simulink model "lqr_pos_control"  (R2021a)
settings: Solver=FixedStepAuto  StartTime=0.0  StopTime=inf  FixedStep=.01  RelTol=1e-3
model workspace (MAT data in the model file):
  SL_ROS_VariableLengthArrays_MaxSizes : object (value not decoded)
values from neighbouring files (symbols this model uses):
  airframe = struct()    [discreteModel_initializer.m]
  Fs = 100    [discreteModel_initializer.m]
  g = 9.81    [discreteModel_initializer.m]
  kLQR = dlqr(lqrDiscrete.A,lqrDiscrete.B,Q,R)    [discreteModel_initializer.m]
  Ts = 1/Fs    (= 0.01)    [discreteModel_initializer.m]
  wiHover = sqrt(((airframe.mass)*9.81)/(4*airframe.Propeller.Ct))    [discreteModel_initializer.m]
undefined symbols (not defined in the file or in its folder): DiscIntNeverNeededParam, Discrete, Gyro_pitch, Gyro_roll, P00, P01, P11, Qkalman, Rkalman, RPM_to_DC, rpmKnown_throttleUnknown, sigbuilder_block, tf1, Time
libraries: robotlib x11, arduinolib x6, sharedtransform x3, simulink x3, ctrlSharedLib x1
(part 2 of 2)

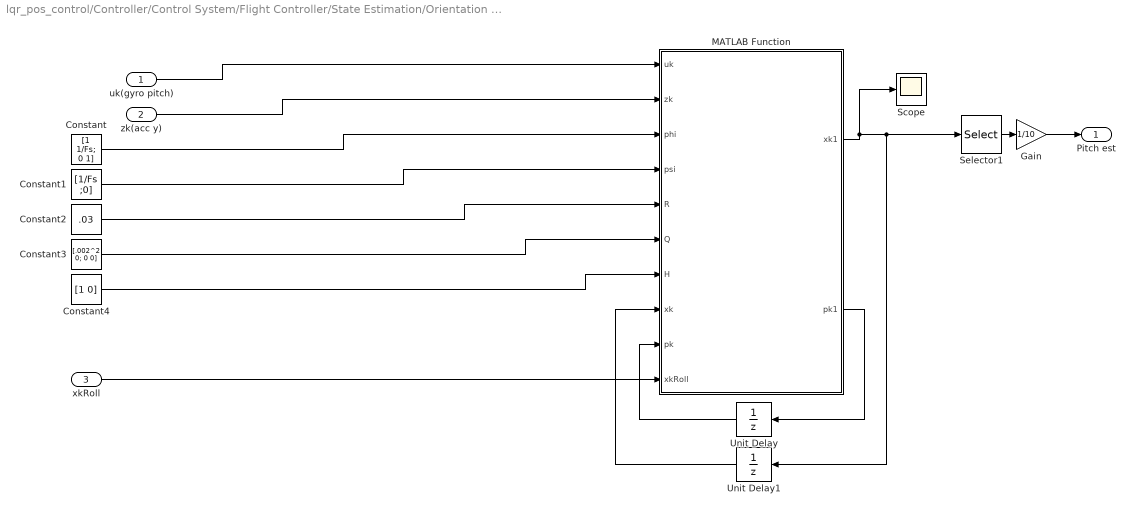
== system lqr_pos_control/Controller/Control System/Flight Controller/State Estimation/Orientation Estimation/Kalman/Kalman Pitch ==
  uk(gyro pitch) : Inport
  zk(acc y) : Inport  Port=2
  xkRoll : Inport  Port=3
  Constant : Constant  Value=[1 1/Fs; 0 1]
  Constant1 : Constant  Value=[1/Fs ;0]
  Constant2 : Constant  Value=.03
  Constant3 : Constant  Value=[.002^2 0; 0 0]
  Constant4 : Constant  Value=[1 0]
  Gain : Gain  Gain=1/10
  MATLAB Function : MATLAB Function  TreatAsAtomicUnit=on
  Scope : Scope
  Selector1 : Selector  InputPortWidth=2  IndexOptions=Index vector (dialog)  Indices=1  OutputSizes=1
  Unit Delay : UnitDelay  InitialCondition=[.5 0; 0 0.01]  SampleTime=-1  HasFrameUpgradeWarning=on
  Unit Delay1 : UnitDelay  InitialCondition=[0;0]  SampleTime=-1  HasFrameUpgradeWarning=on
  Pitch est : Outport
  wires:
  MATLAB Function/1(xk1) -> Scope/1, Unit Delay1/1, Selector1/1
  uk(gyro pitch)/1 -> MATLAB Function/1(uk)
  zk(acc y)/1 -> MATLAB Function/2(zk)
  Constant/1 -> MATLAB Function/3(phi)
  Constant1/1 -> MATLAB Function/4(psi)
  Constant2/1 -> MATLAB Function/5(R)
  Constant3/1 -> MATLAB Function/6(Q)
  Constant4/1 -> MATLAB Function/7(H)
  Selector1/1 -> Gain/1
  Gain/1 -> Pitch est/1
  xkRoll/1 -> MATLAB Function/10(xkRoll)
  MATLAB Function/2(pk1) -> Unit Delay/1
  Unit Delay/1 -> MATLAB Function/9(pk)
  Unit Delay1/1 -> MATLAB Function/8(xk)

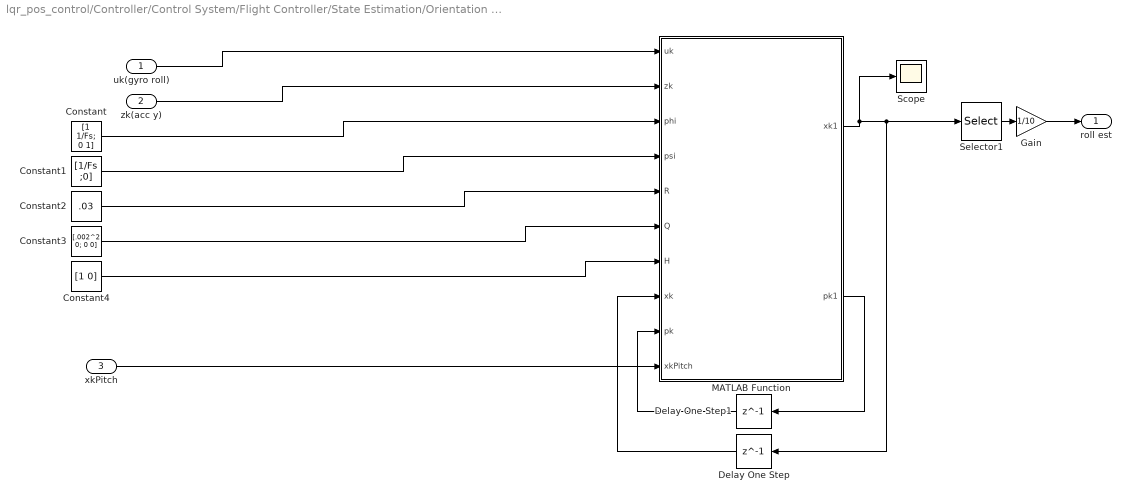
== system lqr_pos_control/Controller/Control System/Flight Controller/State Estimation/Orientation Estimation/Kalman/Kalman ROll ==
  uk(gyro roll) : Inport
  zk(acc y) : Inport  Port=2
  xkPitch : Inport  Port=3
  Constant : Constant  Value=[1 1/Fs; 0 1]
  Constant1 : Constant  Value=[1/Fs ;0]
  Constant2 : Constant  Value=.03
  Constant3 : Constant  Value=[.002^2 0; 0 0]
  Constant4 : Constant  Value=[1 0]
  Delay One Step : Delay  DelayLength=1  InitialCondition=[0;0]
  Delay One Step1 : Delay  DelayLength=1  InitialCondition=[.5 0; 0 0.01]
  Gain : Gain  Gain=1/10
  MATLAB Function : MATLAB Function  TreatAsAtomicUnit=on
  Scope : Scope
  Selector1 : Selector  InputPortWidth=2  IndexOptions=Index vector (dialog)  Indices=1  OutputSizes=1
  roll est : Outport
  wires:
  MATLAB Function/1(xk1) -> Scope/1, Selector1/1, Delay One Step/1
  MATLAB Function/2(pk1) -> Delay One Step1/1
  Delay One Step/1 -> MATLAB Function/8(xk)
  Delay One Step1/1 -> MATLAB Function/9(pk)
  uk(gyro roll)/1 -> MATLAB Function/1(uk)
  zk(acc y)/1 -> MATLAB Function/2(zk)
  Constant/1 -> MATLAB Function/3(phi)
  Constant1/1 -> MATLAB Function/4(psi)
  Constant2/1 -> MATLAB Function/5(R)
  Constant3/1 -> MATLAB Function/6(Q)
  Constant4/1 -> MATLAB Function/7(H)
  Selector1/1 -> Gain/1
  Gain/1 -> roll est/1
  xkPitch/1 -> MATLAB Function/10(xkPitch)

== matlab function lqr_pos_control/Controller/Control System/Motor Mixer/Variant Subsystem/Plus Configuration2/MATLAB Function ==
  data: lArm input; controlMatInv output; Ct input; CdProp input
function controlMatInv = fcn(lArm,Ct,CdProp)

controlMat = [Ct Ct Ct Ct;
    0 lArm*Ct 0 -lArm*Ct;
    -lArm*Ct 0 lArm*Ct 0;
    CdProp -CdProp CdProp -CdProp];

invControlMat = [1/(4*Ct),              0, -1/(2*Ct*lArm),  1/(4*CdProp);
1/(4*Ct),  1/(2*Ct*lArm),              0, -1/(4*CdProp);
1/(4*Ct),              0,  1/(2*Ct*lArm),  1/(4*CdProp);
1/(4*Ct), -1/(2*Ct*lArm),              0, -1/(4*CdProp)];


controlMatInv = invControlMat;

== matlab function lqr_pos_control/Controller/Control System/Flight Controller/State Estimation/Orientation Estimation/Madgwick's Complemntary Filter/MATLAB Function ==
  data: a input; qEst output; wB input; dt input; qIn input
function qEst  = fcn(a,wB,dt,qIn)

gain = 0.01;      
%Returns normalized quaternion prediction from angular velocity vector and prev. quaternion
q0 = qIn(1);
q1 = qIn(2);
q2 = qIn(3);
q3 = qIn(4);

% wx_unb = wx - wx_bias
% wy_unb = wy - wy_bias
% wz_unb = wz - wz_bias
wx_unb = wB(2);
wy_unb = wB(1);
wz_unb = wB(3);


q0_pred = q0 + 0.5 * dt * (wx_unb * q1 + wy_unb * q2 + wz_unb * q3);
q1_pred = q1 + 0.5 * dt * (-wx_unb * q0 - wy_unb * q3 + wz_unb * q2);
q2_pred = q2 + 0.5 * dt * (wx_unb * q3 - wy_unb * q0 - wz_unb * q1);
q3_pred = q3 + 0.5 * dt * (-wx_unb * q2 + wy_unb * q1 - wz_unb * q0);

qOut = [q0_pred, q1_pred, q2_pred, q3_pred];

qPredict = qOut / norm(qOut);


a = a / norm(a);

% % % % % % Acc reading rotated into the world frame by the inverse predicted quaternion (predicted gravity)
% % % % % % gx, gy, gz = self.quatRotate(a[0], a[1], a[2], quat[0], -quat[1], -quat[2],
% % % % % %                         -quat[3])
% % % % % 
% % % % % 

q0 = qPredict(1);
q1 = -qPredict(2);
q2 = -qPredict(3);
q3 = -qPredict(4);
x = a(2);
y = a(1);
z = -a(3);

gx = (q0 * q0 + q1 * q1 - q2 * q2 - q3 * q3) * x + 2 * (q1 * q2 - q0 * q3) * y + 2 * (q1 * q3 + q0 * q2) * z;
gy = 2 * (q1 * q2 + q0 * q3) * x + (q0 * q0 - q1 * q1 + q2 * q2 - q3 * q3) * y + 2 * (q2 * q3 - q0 * q1) * z;
gz = 2 * (q1 * q3 - q0 * q2) * x + 2 * (q2 * q3 + q0 * q1) * y + (q0 * q0 - q1 * q1 - q2 * q2 + q3 * q3) * z;

% % % % % 
% % % gx = a(2);
% % % gy = a(1);
% % % gz = -a(3);
dq0 = sqrt((gz + 1) * .5);
dq1 = -gy / (2 * dq0);
dq2 = gx / (2 * dq0);
dq3 = 0;

dquat = [dq0, dq1, dq2, dq3];


%scale and smooth quaternion
angle = acos(dquat(1));
if dquat(1) < 0
    angle = acos(dquat(1));
    A = sin(angle * (1 - gain)) / sin(angle);
    B = sin(angle * gain) / sin(angle);
    dq0 = A + B * dquat(1);
    dq1 = B * dquat(2);
    dq2 = B * dquat(3);
    dq3 = B * dquat(4);

else 
    dq0 = (1 - gain) + gain * dquat(1);
    dq1 = gain * dquat(2);
    dq2 = gain * dquat(3);
    dq3 = gain * dquat(4);
end
quatOut = [dq0, dq1, dq2, dq3];
qscale = quatOut / norm(quatOut);


a = qPredict;
b = qscale;
ab = zeros(4,1);
ab(1) = dot(a(1), b(1)) - dot(a(2), b(2)) - dot(a(3), b(3)) - dot(a(4), b(4));
ab(2) = dot(a(1), b(2)) + dot(a(2), b(1)) + dot(a(3), b(4)) - dot(a(4), b(3));
ab(3) = dot(a(1), b(3)) - dot(a(2), b(4)) + dot(a(3), b(1)) + dot(a(4), b(2));
ab(4) = dot(a(1), b(4)) + dot(a(2), b(3)) - dot(a(3), b(2)) + dot(a(4), b(1));
qEst = ab;
if sum(a)~=0 
    qEst = qEst / norm(qEst);
else
    qEst = [1 0 0 0]';
end
    


% % % % % 
% % % % %         deltaACC = self.correctAcc(currAccel, quatPredict)
% % % % % 
% % % % %         # alpha = getAdaptiveGain(gain_acc_, ax, ay, az)
% % % % %         alpha = 0.01
% % % % % 
% % % % %         # Returns normalized quaternion
% % % % %         deltaqScale = self.scaleQuat(self.epsilon, alpha, deltaACC)
% % % % % 
% % % % %         self.qInit = self.quatProd(quatPredict, deltaqScale)

== matlab function lqr_pos_control/Controller/Control System/Flight Controller/State Estimation/Orientation Estimation/Kalman/Kalman Pitch/MATLAB Function ==
  data: uk input; xk1 output; zk input; pk1 output; phi input; psi input; R input; Q input; H input; xk input; pk input; xkRoll input
function [xk1,pk1] = fcn(uk,zk,phi,psi,R,Q,H,xk,pk,xkRoll)
xk1Minus = phi*xk+psi*uk(1);
pk1Minus = phi*pk*phi'+Q;
xk1Minus(1) = xk1Minus(1)+xkRoll*sin(uk(2)*.0000013323);
% xk1Minus(1) = xk1Minus(1);
S = H'*pk1Minus*H+R;
K = pk1Minus*H/S;
xk1 = xk1Minus+K*(zk-H'*xk1Minus);
pk1 = (eye(2)-K*H')*pk1Minus;

== matlab function lqr_pos_control/Controller/Control System/Flight Controller/State Estimation/Orientation Estimation/calPoly Kalman/MATLAB Function ==
  data: Accel_output input; y output; Gyro_output input; IC input; P00 input; P01 input; P11 input; P00 output; P01 output; P11 output; dt input; Q input; R input
function [y,P00,P01,P11] = fcn(Accel_output,Gyro_output,IC,P00,P01,P11,dt,Q,R)
Accel_output = [-Accel_output(1),Accel_output(2),-Accel_output(3)];
Gyro_output = [-Gyro_output(1) Gyro_output(2) Gyro_output(3)];
Predicted_pitch = IC(1);
Predicted_roll = IC(2);
angle_z = IC(3);
Accel_output = Accel_output;
Accel_pitch = atan2((Accel_output(2)),...
     (Accel_output(3)));
 

Predicted_pitch = Predicted_pitch + ((Gyro_output(1))) * dt;

Accel_roll = atan2((Accel_output(1) ),...
    (Accel_output(3)));

Predicted_roll = Predicted_roll - ((Gyro_output(2))) * dt; 


P00 = P00+ dt * (2 * P01 + dt * P11); %// Projected error covariance terms from derivation result: Time Update step 2
P01 = P01+ dt * P11; %// Projected error covariance terms from derivation result: Time Update step 2
P00 = P00+ dt * Q; %// Projected error covariance terms from derivation result: Time Update step 2
P11 = P11+ dt * Q; %// Projected error covariance terms from derivation result: Time Update step 2
Kk0 = P00 / (P00 + R); %// Measurement Update step 1
Kk1 = P01 / (P01 + R); %// Measurement Update step 1
Predicted_pitch = Predicted_pitch+ (Accel_pitch - Predicted_pitch) * Kk0; %// Measurement Update step 2
Predicted_roll = Predicted_roll+ (Accel_roll - Predicted_roll) * Kk0; %// Measurement Update step 2
P00 = P00*(1 - Kk0); %// Measurement Update step 3
P01 = P01*(1 - Kk1); %// Measurement Update step 3
P11 = P11- Kk1 * P01; %// Measurement Update step 3
alpha = 0.98;
angle_z = angle_z+Gyro_output(3)*dt;

y = [Predicted_pitch,Predicted_roll,angle_z]';

== matlab function lqr_pos_control/Controller/Control System/Flight Controller/State Estimation/Orientation Estimation/Kalman/Kalman ROll/MATLAB Function ==
  data: uk input; xk1 output; zk input; pk1 output; phi input; psi input; R input; Q input; H input; xk input; pk input; xkPitch input
function [xk1,pk1] = fcn(uk,zk,phi,psi,R,Q,H,xk,pk,xkPitch)
xk1Minus = phi*xk+psi*uk(1);
pk1Minus = phi*pk*phi'+Q;
xk1Minus(1) = xk1Minus(1)-xkPitch*sin(uk(2)*.0000013323);
% xk1Minus(1) = xk1Minus(1);
S = H'*pk1Minus*H+R;
K = pk1Minus*H*inv(S);
xk1 = xk1Minus+K*(zk-H'*xk1Minus);
pk1 = (eye(2)-K*H')*pk1Minus;

== matlab function lqr_pos_control/Controller/Control System/Motor Mixer/Variant Subsystem/Plus Configuration/MATLAB Function ==
  data: lArm input; controlMatInv output; Ct input; CdProp input
function controlMatInv = fcn(lArm,Ct,CdProp)
controlMat = [Ct Ct Ct Ct;
    0 -lArm*Ct 0 lArm*Ct;
    -lArm*Ct 0 lArm*Ct 0;
    CdProp -CdProp CdProp -CdProp];


invControlMat = [1/(4*Ct),0, -1/(2*Ct*lArm), 1/(4*CdProp);
    1/(4*Ct), -1/(2*Ct*lArm),           0, -1/(4*CdProp);
    1/(4*Ct),           0,  1/(2*Ct*lArm),  1/(4*CdProp);
    1/(4*Ct),  1/(2*Ct*lArm),           0, -1/(4*CdProp)];



controlMatInv = invControlMat;

== matlab function lqr_pos_control/Controller/Control System/Motor Mixer/Variant Subsystem/X Configuration/MATLAB Function ==
  data: lArm input; controlMatInv output; Ct input; CdProp input
function controlMatInv = fcn(lArm,Ct,CdProp)
controlMat = [Ct Ct Ct Ct;
    lArm*Ct -lArm*Ct -lArm*Ct lArm*Ct;
    -lArm*Ct -lArm*Ct lArm*Ct lArm*Ct;
    CdProp -CdProp CdProp -CdProp];


invControlMat = [1/(4*Ct),  1/(4*Ct*lArm), -1/(4*Ct*lArm),  1/(4*CdProp);
1/(4*Ct), -1/(4*Ct*lArm), -1/(4*Ct*lArm), -1/(4*CdProp);
1/(4*Ct), -1/(4*Ct*lArm),  1/(4*Ct*lArm),  1/(4*CdProp);
1/(4*Ct),  1/(4*Ct*lArm),  1/(4*Ct*lArm), -1/(4*CdProp)];
controlMatInv = invControlMat;

== stateflow chart lqr_pos_control/Controller/autopilot ==
  settings: updateMethod=DISCRETE  executeAtInitialization=1
  state NormalFlight
    state arm
      entry,during:
      stateCmd = zeros(12,1);
      motor_arm_flag = 0;
    state TakeoffClimb
      entry,during:
      stateCmd = takeoffCmd;
      motor_arm_flag = 1;
    state nav
      entry,during:
      stateCmd = posControl + trimHover;
    state AltitudeHold
      entry,during:
      stateCmd = trimHover;
    state land
      entry,during:
      stateCmd = zeros(12,1);
    note: This flowchart tells the controller to increase z velocity until the switch is turned off
    state disarm
      entry,during:
      stateCmd = zeros(12,1);
      motor_arm_flag = 0;
    (default) -> (junction 411)
    (junction 411) -> arm
    disarm -> TakeoffClimb : [takeoffFlag==1]
    arm -> TakeoffClimb : [takeoffFlag==1]
    TakeoffClimb -> AltitudeHold : [abs(estimatedStates.z- takeoffCmd(7))<=.1 &&...
        |  abs(estimatedStates.z_dot) <= .1]{...
        | hoverFlag = true; trimHover = takeoffCmd;}
    AltitudeHold -> nav [order 2] : after(5,sec)[hoverFlag==true && takeoffFlag == 1]{i = i+1}
    nav -> AltitudeHold [order 2] : after(5,sec)
    nav -> AltitudeHold [order 3] : [i == 3]{hoverFlag = false;}
    nav -> AltitudeHold [order 1] : [takeoffFlag == 0]
    AltitudeHold -> land [order 1] : [takeoffFlag == 0 && abs(estimatedStates.z) <= abs(trimHover(7))+.1...
        | && abs(estimatedStates.z_dot)<=.1...
        | && abs(estimatedStates.x_dot)<=.1...
        | && abs(estimatedStates.y_dot)<=.1]
    land -> disarm : after(3,sec)[abs(estimatedStates.z)<=.05]
  (default) -> NormalFlight
  data: estimatedStates input Bus: stateCommand; takeoffCmd input double; takeoffFlag input; stateCmd output double; trimHover local double =zeros(12,1); posControl input; hoverFlag local boolean =false; motor_arm_flag output; i local =0

== matlab function lqr_pos_control/apply motor_speed/MATLAB Function ==
  data: Bus input; msg output Bus: SL_Bus_lqr_pos_control_mav_msgs_Actuators; angVel input
function msg = fcn(Bus,angVel)
% Bus.AngularVelocities = [angVel(3); angVel(2); angVel(1); angVel(4)];
Bus.AngularVelocities = angVel;
Bus.AngularVelocities_SL_Info.CurrentLength = uint32(4);
msg = Bus;
